simulink model "StewartPlatform"  (R2020a)
settings: Solver=VariableStepAuto  StartTime=0.1  StopTime=35  FixedStep=0.01  MaxStep=0.01  RelTol=1e-3  EnableMultiTasking=on
values from neighbouring files (symbols this model uses):
  Arm_Wrap = 0.75    [ParamLibrary.sldd]
  BaseArm_Wrap = 0.6    [ParamLibrary.sldd]
undefined symbols (not defined in the file or in its folder): X, Y, Z
libraries: sm_lib x122, nesl_utility x32
(part 5 of 5)

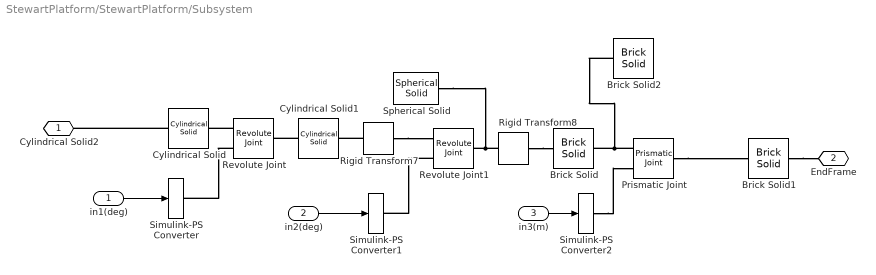
== system StewartPlatform/StewartPlatform/Subsystem ==
  in1(deg) : Inport
  in2(deg) : Inport  Port=2
  in3(m) : Inport  Port=3
  Brick Solid : sm_lib/Body Elements/Brick Solid  GraphicAmbientColor=[0.15 0.15 0.15 1.0]  BasedOnType=Density  BrickDimensions=[0.1 0.05 0.5]  BrickDimensionUnits=m  CenterOfMass=[0 0 0]  CenterOfMassUnits=m  GraphicDiffuseColor=[0.5 0.5 0.5]  Density=1000  DensityUnits=kg/m^3  DoExposeReferenceFrame=off  GraphicEmissiveColor=[0.0 0.0 0.0 1.0]  ExportEntireGeometry=off  SerializedFrames=<Frames><Frame><Id>Frame1</Id><Value><Name>F1</Name><Origin><Source>GeometricFeature</Source><FeatureName>-z surface</FeatureName></Origin><PrimaryAxis><DefinedDirection>+Z</DefinedDirection><Source>ReferenceFrame</Source><SourceDirection>+Z</SourceDirection><FeatureName></FeatureName></PrimaryAxis><SecondaryAxis><DefinedDirection>+X</DefinedDirection><Source>ReferenceFrame</Source><SourceDirection>+X</SourceDirection><FeatureName></FeatureName></SecondaryAxis></Value></Frame><Frame><Id>Frame2</Id><Value><Name>F2</Name><Origin><Source>GeometricFeature</Source><FeatureName>+z surface</FeatureName></Origin><PrimaryAxis><DefinedDirection>+Z</DefinedDirection><Source>ReferenceFrame</Source><SourceDirection>+Z</SourceDirection><FeatureName></FeatureName></PrimaryAxis><SecondaryAxis><DefinedDirection>+X</DefinedDirection><Source>ReferenceFrame</Source><SourceDirection>+X</SourceDirection><FeatureName></FeatureName></SecondaryAxis></Value></Frame></Frames>  MarkerShape=Sphere  MarkerSize=10  GraphicType=FromGeometry  InertiaType=CalculateFromGeometry  Mass=1  MassUnits=kg  MomentsOfInertia=[1 1 1]  MomentsOfInertiaUnits=kg*m^2  GraphicOpacity=1.0  ProductsOfInertia=[0 0 0]  ProductsOfInertiaUnits=kg*m^2  GraphicShininess=75  GraphicSpecularColor=[0.5 0.5 0.5 1.0]  GraphicVisPropType=SimpleVisualProperties
  Brick Solid1 : sm_lib/Body Elements/Brick Solid  GraphicAmbientColor=[0.15 0.15 0.15 1.0]  BasedOnType=Density  BrickDimensions=[0.075 0.02 1]  BrickDimensionUnits=m  CenterOfMass=[0 0 0]  CenterOfMassUnits=m  GraphicDiffuseColor=[0.5 0.5 0.5]  Density=1000  DensityUnits=kg/m^3  DoExposeReferenceFrame=off  GraphicEmissiveColor=[0.0 0.0 0.0 1.0]  ExportEntireGeometry=off  SerializedFrames=<Frames><Frame><Id>Frame1</Id><Value><Name>F1</Name><Origin><Source>GeometricFeature</Source><FeatureName>-z surface</FeatureName></Origin><PrimaryAxis><DefinedDirection>+Z</DefinedDirection><Source>ReferenceFrame</Source><SourceDirection>+Z</SourceDirection><FeatureName></FeatureName></PrimaryAxis><SecondaryAxis><DefinedDirection>+X</DefinedDirection><Source>ReferenceFrame</Source><SourceDirection>+X</SourceDirection><FeatureName></FeatureName></SecondaryAxis></Value></Frame><Frame><Id>Frame2</Id><Value><Name>F2</Name><Origin><Source>GeometricFeature</Source><FeatureName>+z surface</FeatureName></Origin><PrimaryAxis><DefinedDirection>+Z</DefinedDirection><Source>ReferenceFrame</Source><SourceDirection>+Z</SourceDirection><FeatureName></FeatureName></PrimaryAxis><SecondaryAxis><DefinedDirection>+X</DefinedDirection><Source>ReferenceFrame</Source><SourceDirection>+X</SourceDirection><FeatureName></FeatureName></SecondaryAxis></Value></Frame></Frames>  MarkerShape=Sphere  MarkerSize=10  GraphicType=FromGeometry  InertiaType=CalculateFromGeometry  Mass=1  MassUnits=kg  MomentsOfInertia=[1 1 1]  MomentsOfInertiaUnits=kg*m^2  GraphicOpacity=1.0  ProductsOfInertia=[0 0 0]  ProductsOfInertiaUnits=kg*m^2  GraphicShininess=75  GraphicSpecularColor=[0.5 0.5 0.5 1.0]  GraphicVisPropType=SimpleVisualProperties
  Brick Solid2 : sm_lib/Body Elements/Brick Solid  GraphicAmbientColor=[0.15 0.15 0.15 1.0]  BasedOnType=Density  BrickDimensions=[0.1 0.05 1.5]  BrickDimensionUnits=m  CenterOfMass=[0 0 0]  CenterOfMassUnits=m  GraphicDiffuseColor=[0.5 0.5 0.5]  Density=1000  DensityUnits=kg/m^3  DoExposeReferenceFrame=off  GraphicEmissiveColor=[0.0 0.0 0.0 1.0]  ExportEntireGeometry=off  SerializedFrames=<Frames><Frame><Id>Frame1</Id><Value><Name>F1</Name><Origin><Source>GeometricFeature</Source><FeatureName>-z surface</FeatureName></Origin><PrimaryAxis><DefinedDirection>+Z</DefinedDirection><Source>ReferenceFrame</Source><SourceDirection>+Z</SourceDirection><FeatureName></FeatureName></PrimaryAxis><SecondaryAxis><DefinedDirection>+X</DefinedDirection><Source>ReferenceFrame</Source><SourceDirection>+X</SourceDirection><FeatureName></FeatureName></SecondaryAxis></Value></Frame></Frames>  MarkerShape=Sphere  MarkerSize=10  GraphicType=FromGeometry  InertiaType=CalculateFromGeometry  Mass=1  MassUnits=kg  MomentsOfInertia=[1 1 1]  MomentsOfInertiaUnits=kg*m^2  GraphicOpacity=1.0  ProductsOfInertia=[0 0 0]  ProductsOfInertiaUnits=kg*m^2  GraphicShininess=75  GraphicSpecularColor=[0.5 0.5 0.5 1.0]  GraphicVisPropType=SimpleVisualProperties
  Cylindrical Solid : sm_lib/Body Elements/Cylindrical Solid  GraphicAmbientColor=[0.15 0.15 0.15 1.0]  BasedOnType=Density  CenterOfMass=[0 0 0]  CenterOfMassUnits=m  GraphicDiffuseColor=[0.5 0.5 0.5]  CylinderLength=0.2  CylinderLengthUnits=m  CylinderRadius=0.3  CylinderRadiusUnits=m  Density=1000  DensityUnits=kg/m^3  DoExposeReferenceFrame=off  GraphicEmissiveColor=[0.0 0.0 0.0 1.0]  ExportEntireGeometry=off  SerializedFrames=<Frames><Frame><Id>Frame1</Id><Value><Name>F1</Name><Origin><Source>GeometricFeature</Source><FeatureName>bottom surface</FeatureName></Origin><PrimaryAxis><DefinedDirection>+Z</DefinedDirection><Source>ReferenceFrame</Source><SourceDirection>+Z</SourceDirection><FeatureName></FeatureName></PrimaryAxis><SecondaryAxis><DefinedDirection>+X</DefinedDirection><Source>ReferenceFrame</Source><SourceDirection>+X</SourceDirection><FeatureName></FeatureName></SecondaryAxis></Value></Frame><Frame><Id>Frame2</Id><Value><Name>F2</Name><Origin><Source>GeometricFeature</Source><FeatureName>top surface</FeatureName></Origin><PrimaryAxis><DefinedDirection>+Z</DefinedDirection><Source>ReferenceFrame</Source><SourceDirection>+Z</SourceDirection><FeatureName></FeatureName></PrimaryAxis><SecondaryAxis><DefinedDirection>+X</DefinedDirection><Source>ReferenceFrame</Source><SourceDirection>+X</SourceDirection><FeatureName></FeatureName></SecondaryAxis></Value></Frame></Frames>  MarkerShape=Sphere  MarkerSize=10  GraphicType=FromGeometry  InertiaType=CalculateFromGeometry  Mass=1  MassUnits=kg  MomentsOfInertia=[1 1 1]  MomentsOfInertiaUnits=kg*m^2  GraphicOpacity=1.0  ProductsOfInertia=[0 0 0]  ProductsOfInertiaUnits=kg*m^2  GraphicShininess=75  GraphicSpecularColor=[0.5 0.5 0.5 1.0]  GraphicVisPropType=SimpleVisualProperties
  Cylindrical Solid1 : sm_lib/Body Elements/Cylindrical Solid  GraphicAmbientColor=[0.15 0.15 0.15 1.0]  BasedOnType=Density  CenterOfMass=[0 0 0]  CenterOfMassUnits=m  GraphicDiffuseColor=[0.5 0.5 0.5]  CylinderLength=0.4  CylinderLengthUnits=m  CylinderRadius=0.1  CylinderRadiusUnits=m  Density=1000  DensityUnits=kg/m^3  DoExposeReferenceFrame=off  GraphicEmissiveColor=[0.0 0.0 0.0 1.0]  ExportEntireGeometry=off  SerializedFrames=<Frames><Frame><Id>Frame1</Id><Value><Name>F1</Name><Origin><Source>GeometricFeature</Source><FeatureName>bottom surface</FeatureName></Origin><PrimaryAxis><DefinedDirection>+Z</DefinedDirection><Source>ReferenceFrame</Source><SourceDirection>+Z</SourceDirection><FeatureName></FeatureName></PrimaryAxis><SecondaryAxis><DefinedDirection>+X</DefinedDirection><Source>ReferenceFrame</Source><SourceDirection>+X</SourceDirection><FeatureName></FeatureName></SecondaryAxis></Value></Frame><Frame><Id>Frame2</Id><Value><Name>F2</Name><Origin><Source>GeometricFeature</Source><FeatureName>top surface</FeatureName></Origin><PrimaryAxis><DefinedDirection>+Z</DefinedDirection><Source>ReferenceFrame</Source><SourceDirection>+Z</SourceDirection><FeatureName></FeatureName></PrimaryAxis><SecondaryAxis><DefinedDirection>+X</DefinedDirection><Source>ReferenceFrame</Source><SourceDirection>+X</SourceDirection><FeatureName></FeatureName></SecondaryAxis></Value></Frame></Frames>  MarkerShape=Sphere  MarkerSize=10  GraphicType=FromGeometry  InertiaType=CalculateFromGeometry  Mass=1  MassUnits=kg  MomentsOfInertia=[1 1 1]  MomentsOfInertiaUnits=kg*m^2  GraphicOpacity=1.0  ProductsOfInertia=[0 0 0]  ProductsOfInertiaUnits=kg*m^2  GraphicShininess=75  GraphicSpecularColor=[0.5 0.5 0.5 1.0]  GraphicVisPropType=SimpleVisualProperties
  Prismatic Joint : sm_lib/Joints/Prismatic Joint  JointMode=Normal  SenseConstraintForce=off  SenseConstraintForceX=off  SenseConstraintForceY=off  SenseConstraintForceZ=off  SenseConstraintTorque=off  SenseConstraintTorqueX=off  SenseConstraintTorqueY=off  SenseConstraintTorqueZ=off  SenseTotalForce=off  SenseTotalForceX=off  SenseTotalForceY=off  SenseTotalForceZ=off  SenseTotalTorque=off  SenseTotalTorqueX=off  SenseTotalTorqueY=off  SenseTotalTorqueZ=off  CompositeWrenchDir=FollowerOnBase  CompositeWrenchFrame=BaseFrame  EquilibriumPosition=0  EquilibriumPositionUnits=m  SpringStiffness=0  SpringStiffnessUnits=N/m  DampingCoefficient=0  DampingCoefficientUnits=N/(m/s)  TorqueActuationMode=ComputedTorque  MotionActuationMode=InputMotion  SensePosition=off  SenseVelocity=off  SenseAcceleration=off  SenseTorqueForce=off  SenseLowerLimitTorqueForce=off  SenseUpperLimitTorqueForce=off  LowerLimitSpecify=on  LowerLimitBound=Arm_LowLimit  LowerLimitBoundUnits=m  LowerLimitStiffness=1e6  LowerLimitStiffnessUnits=N/m  LowerLimitDamping=1e3  LowerLimitDampingUnits=N/(m/s)  LowerLimitTransitionRegionWidth=1e-4  LowerLimitTransitionRegionWidthUnits=m  UpperLimitSpecify=on  UpperLimitBound=Arm_HighLimit  UpperLimitBoundUnits=m  UpperLimitStiffness=1e6  UpperLimitStiffnessUnits=N/m  UpperLimitDamping=1e3  UpperLimitDampingUnits=N/(m/s)  UpperLimitTransitionRegionWidth=1e-4  UpperLimitTransitionRegionWidthUnits=m  PositionTargetSpecify=off  PositionTargetPriority=Low  PositionTargetValue=0.8  PositionTargetValueUnits=m  VelocityTargetSpecify=off  VelocityTargetPriority=High  VelocityTargetValue=0  VelocityTargetValueUnits=m/s
  Revolute Joint : sm_lib/Joints/Revolute Joint  JointMode=Normal  SenseConstraintForce=off  SenseConstraintForceX=off  SenseConstraintForceY=off  SenseConstraintForceZ=off  SenseConstraintTorque=off  SenseConstraintTorqueX=off  SenseConstraintTorqueY=off  SenseConstraintTorqueZ=off  SenseTotalForce=off  SenseTotalForceX=off  SenseTotalForceY=off  SenseTotalForceZ=off  SenseTotalTorque=off  SenseTotalTorqueX=off  SenseTotalTorqueY=off  SenseTotalTorqueZ=off  CompositeWrenchDir=FollowerOnBase  CompositeWrenchFrame=BaseFrame  EquilibriumPosition=0  EquilibriumPositionUnits=deg  SpringStiffness=0  SpringStiffnessUnits=N*m/deg  DampingCoefficient=0  DampingCoefficientUnits=N*m/(deg/s)  TorqueActuationMode=ComputedTorque  MotionActuationMode=InputMotion  SensePosition=off  SenseVelocity=off  SenseAcceleration=off  SenseTorqueForce=off  SenseLowerLimitTorqueForce=off  SenseUpperLimitTorqueForce=off  LowerLimitSpecify=off  LowerLimitBound=-90  LowerLimitBoundUnits=deg  LowerLimitStiffness=1e4  LowerLimitStiffnessUnits=N*m/deg  LowerLimitDamping=10  LowerLimitDampingUnits=N*m/(deg/s)  LowerLimitTransitionRegionWidth=0.1  LowerLimitTransitionRegionWidthUnits=deg  UpperLimitSpecify=off  UpperLimitBound=90  UpperLimitBoundUnits=deg  UpperLimitStiffness=1e4  UpperLimitStiffnessUnits=N*m/deg  UpperLimitDamping=10  UpperLimitDampingUnits=N*m/(deg/s)  UpperLimitTransitionRegionWidth=0.1  UpperLimitTransitionRegionWidthUnits=deg  PositionTargetSpecify=off  PositionTargetPriority=High  PositionTargetValue=0  PositionTargetValueUnits=deg  VelocityTargetSpecify=off  VelocityTargetPriority=High  VelocityTargetValue=0  VelocityTargetValueUnits=deg/s
  Revolute Joint1 : sm_lib/Joints/Revolute Joint  JointMode=Normal  SenseConstraintForce=off  SenseConstraintForceX=off  SenseConstraintForceY=off  SenseConstraintForceZ=off  SenseConstraintTorque=off  SenseConstraintTorqueX=off  SenseConstraintTorqueY=off  SenseConstraintTorqueZ=off  SenseTotalForce=off  SenseTotalForceX=off  SenseTotalForceY=off  SenseTotalForceZ=off  SenseTotalTorque=off  SenseTotalTorqueX=off  SenseTotalTorqueY=off  SenseTotalTorqueZ=off  CompositeWrenchDir=FollowerOnBase  CompositeWrenchFrame=BaseFrame  EquilibriumPosition=0  EquilibriumPositionUnits=deg  SpringStiffness=0  SpringStiffnessUnits=N*m/deg  DampingCoefficient=0  DampingCoefficientUnits=N*m/(deg/s)  TorqueActuationMode=ComputedTorque  MotionActuationMode=InputMotion  SensePosition=off  SenseVelocity=off  SenseAcceleration=off  SenseTorqueForce=off  SenseLowerLimitTorqueForce=off  SenseUpperLimitTorqueForce=off  LowerLimitSpecify=off  LowerLimitBound=-90  LowerLimitBoundUnits=deg  LowerLimitStiffness=1e4  LowerLimitStiffnessUnits=N*m/deg  LowerLimitDamping=10  LowerLimitDampingUnits=N*m/(deg/s)  LowerLimitTransitionRegionWidth=0.1  LowerLimitTransitionRegionWidthUnits=deg  UpperLimitSpecify=off  UpperLimitBound=90  UpperLimitBoundUnits=deg  UpperLimitStiffness=1e4  UpperLimitStiffnessUnits=N*m/deg  UpperLimitDamping=10  UpperLimitDampingUnits=N*m/(deg/s)  UpperLimitTransitionRegionWidth=0.1  UpperLimitTransitionRegionWidthUnits=deg  PositionTargetSpecify=off  PositionTargetPriority=High  PositionTargetValue=0  PositionTargetValueUnits=deg  VelocityTargetSpecify=off  VelocityTargetPriority=High  VelocityTargetValue=0  VelocityTargetValueUnits=deg/s
  Rigid Transform7 : sm_lib/Frames and Transforms/Rigid Transform  TranslationMethod=None  TranslationStandardOffset=0  TranslationLengthUnit=m  TranslationStandardAxis=+Z  TranslationCartesianOffset=[0 0 0]  TranslationROffset=1  TranslationROffsetUnits=m  TranslationZOffset=0  TranslationZOffsetUnits=m  TranslationThetaOffset=0  TranslationThetaOffsetUnits=deg  RotationMethod=StandardAxis  RotationAngleUnits=deg  RotationStandardAxis=+Y  RotationAngle=90.0  RotationArbitraryAxis=[0 0 1]  FollAlignAxisA=+X  BaseAlignAxisA=+Y  FollAlignAxisB=+Y  BaseAlignAxisB=+Z  RotationSequenceAxes=FollowerAxes  RotationSequence=XYX  RotationSequenceAngles=[0 0 0]  RotationSequenceAnglesUnits=deg  RotationMatrix=[1 0 0; 0 1 0; 0 0 1]
  Rigid Transform8 : sm_lib/Frames and Transforms/Rigid Transform  TranslationMethod=None  TranslationStandardOffset=0  TranslationLengthUnit=m  TranslationStandardAxis=+Z  TranslationCartesianOffset=[0 0 0]  TranslationROffset=1  TranslationROffsetUnits=m  TranslationZOffset=0  TranslationZOffsetUnits=m  TranslationThetaOffset=0  TranslationThetaOffsetUnits=deg  RotationMethod=StandardAxis  RotationAngleUnits=deg  RotationStandardAxis=+Y  RotationAngle=90.0  RotationArbitraryAxis=[0 0 1]  FollAlignAxisA=+X  BaseAlignAxisA=+Y  FollAlignAxisB=+Y  BaseAlignAxisB=+Z  RotationSequenceAxes=FollowerAxes  RotationSequence=XYX  RotationSequenceAngles=[0 0 0]  RotationSequenceAnglesUnits=deg  RotationMatrix=[1 0 0; 0 1 0; 0 0 1]
  Simulink-PS Converter : nesl_utility/Simulink-PS Converter  PhysicalDomain=network_engine_domain  SubClassName=ps_input  LeftPortType=input  RightPortType=output  PseudoPeriodic=off  Frequencies=[]  NoiseDistribution=none  NoiseParameters=[]  Unit=1  AffineConversion=off  FilteringAndDerivatives=filter  SimscapeFilterOrder=2  InputFilterTimeConstant=0.001  UdotUserProvided=0
  Simulink-PS Converter1 : nesl_utility/Simulink-PS Converter  PhysicalDomain=network_engine_domain  SubClassName=ps_input  LeftPortType=input  RightPortType=output  PseudoPeriodic=off  Frequencies=[]  NoiseDistribution=none  NoiseParameters=[]  Unit=1  AffineConversion=off  FilteringAndDerivatives=filter  SimscapeFilterOrder=2  InputFilterTimeConstant=0.001  UdotUserProvided=0
  Simulink-PS Converter2 : nesl_utility/Simulink-PS Converter  PhysicalDomain=network_engine_domain  SubClassName=ps_input  LeftPortType=input  RightPortType=output  PseudoPeriodic=off  Frequencies=[]  NoiseDistribution=none  NoiseParameters=[]  Unit=1  AffineConversion=off  FilteringAndDerivatives=filter  SimscapeFilterOrder=2  InputFilterTimeConstant=0.001  UdotUserProvided=0
  Spherical Solid : sm_lib/Body Elements/Spherical Solid  GraphicAmbientColor=[0.15 0.15 0.15 1.0]  BasedOnType=Density  CenterOfMass=[0 0 0]  CenterOfMassUnits=m  GraphicDiffuseColor=[0.5 0.5 0.5]  Density=1000  DensityUnits=kg/m^3  DoExposeReferenceFrame=on  GraphicEmissiveColor=[0.0 0.0 0.0 1.0]  ExportEntireGeometry=off  SerializedExposedGeometries=<ExposedGeometries/>  SerializedFrames=<Frames/>  MarkerShape=Sphere  MarkerSize=10  GraphicType=FromGeometry  InertiaType=CalculateFromGeometry  Mass=1  MassUnits=kg  MomentsOfInertia=[1 1 1]  MomentsOfInertiaUnits=kg*m^2  GraphicOpacity=1.0  ProductsOfInertia=[0 0 0]  ProductsOfInertiaUnits=kg*m^2  GraphicShininess=75  GraphicSpecularColor=[0.5 0.5 0.5 1.0]  SphereRadius=0.1  SphereRadiusUnits=m  GraphicVisPropType=SimpleVisualProperties
  Cylindrical Solid2 : PMIOPort  Side=Left
  EndFrame : PMIOPort  Port=2  Side=Right
  wires:
  in1(deg)/1 -> Simulink-PS Converter/1
  in2(deg)/1 -> Simulink-PS Converter1/1
  in3(m)/1 -> Simulink-PS Converter2/1
  connections:
  Prismatic Joint/LConn1 -- Brick Solid2/LConn1 -- Brick Solid/RConn1
  Rigid Transform7/RConn1 -- Revolute Joint1/LConn1
  Rigid Transform7/LConn1 -- Cylindrical Solid1/RConn1
  Rigid Transform8/LConn1 -- Spherical Solid/RConn1 -- Revolute Joint1/RConn1
  Cylindrical Solid1/LConn1 -- Revolute Joint/RConn1
  Revolute Joint/LConn1 -- Cylindrical Solid/RConn1
  Rigid Transform8/RConn1 -- Brick Solid/LConn1
  Revolute Joint/LConn2 -- Simulink-PS Converter/RConn1
  Revolute Joint1/LConn2 -- Simulink-PS Converter1/RConn1
  Prismatic Joint/RConn1 -- Brick Solid1/LConn1
  Cylindrical Solid/LConn1 -- Cylindrical Solid2/RConn1
  Simulink-PS Converter2/RConn1 -- Prismatic Joint/LConn2
  Brick Solid1/RConn1 -- EndFrame/RConn1

== matlab function StewartPlatform/MATLAB Function1 ==
  data: TF_CA input; alpha output; beita output; dL output
function [alpha,beita,dL] = fcn(TF_CA)
% 原有计算逻辑
TF_CEnd_Static = [1,0.004,0.1,0.17;
                  0.1,-0.07,-1,-1.77;
                  0.0026,1,-0.07,4;
                  0,0,0,1];
L = 0.6;
L1 = 0.5;
L2 = 1;
TF_AEnd = pinv(TF_CA) * TF_CEnd_Static;
x = TF_AEnd(1,4);
y = TF_AEnd(2,4);
z = TF_AEnd(3,4);

dL = sqrt((z-L)^2 + x^2 + y^2) - (L1 + L2); % 更安全的sqrt写法
beita = asin((z-L)/(L1+L2+dL));
alpha = asin(y/( (L1+L2+dL)*cos(beita) )); % 修正分母的括号
end

== matlab function StewartPlatform/TF_Coder ==
  data: RotationMatrix input; X input; TF_Matrix output; Y input; Z input
function TF_Matrix = fcn(RotationMatrix,X, Y, Z)
 T = [
        RotationMatrix(1,1), RotationMatrix(1,2), RotationMatrix(1,3), X;
        RotationMatrix(2,1), RotationMatrix(2,2), RotationMatrix(2,3), Y;
        RotationMatrix(3,1), RotationMatrix(3,2), RotationMatrix(3,3), Z;
        0, 0, 0, 1;
    ];

TF_Matrix = T;

== matlab function StewartPlatform/TF_Coder1 ==
  data: RotationMatrix input; X input; TF_Matrix output; Y input; Z input
function TF_Matrix = fcn(RotationMatrix,X, Y, Z)
 T = [
        RotationMatrix(1,1), RotationMatrix(1,2), RotationMatrix(1,3), X;
        RotationMatrix(2,1), RotationMatrix(2,2), RotationMatrix(2,3), Y;
        RotationMatrix(3,1), RotationMatrix(3,2), RotationMatrix(3,3), Z;
        0, 0, 0, 1;
    ];

TF_Matrix = T;

== matlab function StewartPlatform/TF_Coder ==
  data: RotationMatrix input; X input; TF_Matrix output; Y input; Z input
function TF_Matrix = fcn(RotationMatrix,X, Y, Z)
 T = [
        RotationMatrix(1,1), RotationMatrix(1,2), RotationMatrix(1,3), X;
        RotationMatrix(2,1), RotationMatrix(2,2), RotationMatrix(2,3), Y;
        RotationMatrix(3,1), RotationMatrix(3,2), RotationMatrix(3,3), Z;
        0, 0, 0, 1;
    ];

TF_Matrix = T;

== matlab function StewartPlatform/Controller_SelfFit ==
  data: TF_CB input; TF_BA input; Arm1 output; Arm2 output; Arm3 output; Arm4 output; Arm5 output; Arm6 output; Mode input; Robustness input
function [Arm1, Arm2, Arm3, Arm4, Arm5, Arm6] = fcn(TF_CB,TF_BA,Mode,Robustness)
%Frame_A相对Frame_B初始位姿
TF_BA_Static = [
-0.866  ,-0.5    ,0     ,0 ;    
 0.5    ,-0.866  ,0     ,0 ;
 0      ,0       ,1     ,1.518;
 0      ,0       ,0     ,1    
];
%Frame_B相对Frame_C初始位姿
TF_CB_Static = [
0.866  ,-0.5    ,0     ,0 ;    
 0.5    ,0.866  ,0     ,0 ;
 0      ,0       ,1     ,(1.305+0.6);
 0      ,0       ,0     ,1    
];
TF_CA_Static = TF_CB_Static * TF_BA_Static ;
%A面和B面点坐标
Ra = 0.8;
a1 = [-Ra/2 ; -(3)^(0.5)*Ra/2 ; 0];
a2 = [Ra ; 0 ; 0];
a3 = [-Ra/2 ; (3)^(0.5)*Ra/2 ; 0 ];
Rb = 1;
b1 = [Rb;0;0];
b2 = [Rb/2;(3)^(0.5)*Rb/2;0];
b3 = [-Rb/2;(3)^(0.5)*Rb/2;0];
b4 = [-Rb;0;0];
b5 = [-Rb/2;-(3)^(0.5)*Rb/2;0];
b6 = [Rb/2;-(3)^(0.5)*Rb/2;0];
if Mode == 0
%%上平台完全静止
%求解最上层平台Frame_A相对Frame_B的目标位姿
    TF_BA_Target = pinv(TF_CB) * TF_CA_Static ;
    Arm1 = norm( TF_BA_Target*[a1;1] - [b1;1]  ) - 1.6;
    Arm2 = norm( TF_BA_Target*[a1;1] - [b2;1]  ) - 1.6;
    Arm3 = norm( TF_BA_Target*[a2;1] - [b3;1]  ) - 1.6;
    Arm4 = norm( TF_BA_Target*[a2;1] - [b4;1]  ) - 1.6;
    Arm5 = norm( TF_BA_Target*[a3;1] - [b5;1]  ) - 1.6;
    Arm6 = norm( TF_BA_Target*[a3;1] - [b6;1]  ) - 1.6;
%%上平台自由平滑跟随
elseif Mode == 1
    TF_CA_NOW = TF_CB * TF_BA;
    TF_CA_Target = [
        TF_CA_Static(1,1) , TF_CA_Static(1,2) , TF_CA_Static(1,3) , (TF_CA_Static(1,4)*Robustness + TF_CA_NOW(1,4))/(Robustness+1);
        TF_CA_Static(2,1) , TF_CA_Static(2,2) , TF_CA_Static(2,3) , (TF_CA_Static(2,4)*Robustness + TF_CA_NOW(2,4))/(Robustness+1) ;
        TF_CA_Static(3,1) , TF_CA_Static(3,2) , TF_CA_Static(3,3) , (TF_CA_Static(3,4)*Robustness + TF_CA_NOW(3,4))/(Robustness+1);
        0 ,0 ,0 ,1
    ];
    TF_BA_Target = pinv(TF_CB) * TF_CA_Target;
    Arm1 = norm( TF_BA_Target*[a1;1] - [b1;1]  ) - 1.6;
    Arm2 = norm( TF_BA_Target*[a1;1] - [b2;1]  ) - 1.6;
    Arm3 = norm( TF_BA_Target*[a2;1] - [b3;1]  ) - 1.6;
    Arm4 = norm( TF_BA_Target*[a2;1] - [b4;1]  ) - 1.6;
    Arm5 = norm( TF_BA_Target*[a3;1] - [b5;1]  ) - 1.6;
    Arm6 = norm( TF_BA_Target*[a3;1] - [b6;1]  ) - 1.6;
    
else
Arm1 = 0;
Arm2 = 0;
Arm3 = 0;
Arm4 = 0;
Arm5 = 0;
Arm6 = 0;
end

end

== matlab function StewartPlatform/TF_Coder1 ==
  data: RotationMatrix input; X input; TF_Matrix output; Y input; Z input
function TF_Matrix = fcn(RotationMatrix,X, Y, Z)
 T = [
        RotationMatrix(1,1), RotationMatrix(1,2), RotationMatrix(1,3), X;
        RotationMatrix(2,1), RotationMatrix(2,2), RotationMatrix(2,3), Y;
        RotationMatrix(3,1), RotationMatrix(3,2), RotationMatrix(3,3), Z;
        0, 0, 0, 1;
    ];

TF_Matrix = T;

== matlab function StewartPlatform/Controller_outctrl ==
  data: TF_CB input; Arm1 output; TF_BA input; TF_CA_Static_last input; clock input; Mode input; Arm2 output; Arm3 output; Arm4 output; Arm5 output; Arm6 output; Robustness input; M11 output; M12 output; M13 output; M14 output; M21 output; M22 output; M23 output; M24 output; M31 output; M32 output; M33 output; M34 output
function [Arm1, Arm2, Arm3, Arm4, Arm5, Arm6, M11, M12, M13, M14, M21, M22, M23, M24, M31, M32, M33, M34]  = fcn(TF_CB,TF_BA,TF_CA_Static_last,clock,Mode,Robustness)
%Frame_A相对Frame_B初始位姿
TF_BA_Static = [
-0.866  ,-0.5    ,0     ,0 ;    
 0.5    ,-0.866  ,0     ,0 ;
 0      ,0       ,1     ,1.518;
 0      ,0       ,0     ,1    
];
%Frame_B相对Frame_C初始位姿
TF_CB_Static = [
0.866  ,-0.5    ,0     ,0 ;    
 0.5    ,0.866  ,0     ,0 ;
 0      ,0       ,1     ,(1.305+0.6);
 0      ,0       ,0     ,1    
];
TF_CA_Static = TF_CB_Static * TF_BA_Static ;
%继承上一周期的TF_CA_Static
start_time = 1;
phase = 2;
if clock > start_time
    TF_CA_Static = TF_CA_Static_last;
end

seta = 0.002;
TF_ROT_X = [1,0,0,0;
            0,cos(seta),-sin(seta),0;
            0,sin(seta),cos(seta),0;
            0,0,0,1];
TF_ROT_X_n = [1,0,0,0;
            0,cos(-seta),-sin(-seta),0;
            0,sin(-seta),cos(-seta),0;
            0,0,0,1];
TF_ROT_Y = [cos(seta), 0, sin(seta), 0;
            0, 1, 0, 0;
            -sin(seta), 0, cos(seta), 0;
            0, 0, 0, 1];
TF_ROT_Y_n = [cos(-seta),0,sin(-seta),0;
            0,1,0,0;
            -sin(-seta),0,cos(-seta),0;
            0,0,0,1];
TF_ROT_Z = [cos(seta),-sin(seta),0,0;
            sin(seta),cos(seta),0,0;
            0,0,1,0;
            0,0,0,1;
];
TF_ROT_Z_n = [cos(-seta),-sin(-seta),0,0;
            sin(-seta),cos(-seta),0,0;
            0,0,1,0;
            0,0,0,1;
];
%x轴倾斜
if (start_time<clock)&&(clock<start_time+phase)
    TF_CA_Static = TF_CA_Static * TF_ROT_X_n;   
end
if (start_time+phase<clock)&&(clock<start_time+2*phase)
    TF_CA_Static =  TF_CA_Static * TF_ROT_X;   
end
if (start_time+2*phase<clock)&&(clock<start_time+3*phase)
    TF_CA_Static = TF_CA_Static * TF_ROT_X;   
end
if (start_time+3*phase<clock)&&(clock<start_time+4*phase)
    TF_CA_Static = TF_CA_Static * TF_ROT_X_n;   
end
%y轴倾斜
if (start_time+4*phase<clock)&&(clock<start_time+5*phase)
    TF_CA_Static = TF_CA_Static * TF_ROT_Y_n;   
end
if (start_time+5*phase<clock)&&(clock<start_time+6*phase)
    TF_CA_Static = TF_CA_Static * TF_ROT_Y;   
end
if (start_time+6*phase<clock)&&(clock<start_time+7*phase)
    TF_CA_Static = TF_CA_Static * TF_ROT_Y;   
end
if (start_time+7*phase<clock)&&(clock<start_time+8*phase)
    TF_CA_Static = TF_CA_Static * TF_ROT_Y_n;   
end
%z轴倾斜
if (start_time+8*phase<clock)&&(clock<start_time+9*phase)
    TF_CA_Static = TF_CA_Static * TF_ROT_Z_n;   
end
if (start_time+9*phase<clock)&&(clock<start_time+10*phase)
    TF_CA_Static = TF_CA_Static * TF_ROT_Z;   
end
if (start_time+10*phase<clock)&&(clock<start_time+11*phase)
    TF_CA_Static = TF_CA_Static * TF_ROT_Z;   
end
if (start_time+11*phase<clock)&&(clock<start_time+12*phase)
    TF_CA_Static = TF_CA_Static * TF_ROT_Z_n;   
end


%A面和B面点坐标
Ra = 0.8;
a1 = [-Ra/2 ; -(3)^(0.5)*Ra/2 ; 0];
a2 = [Ra ; 0 ; 0];
a3 = [-Ra/2 ; (3)^(0.5)*Ra/2 ; 0 ];
Rb = 1;
b1 = [Rb;0;0];
b2 = [Rb/2;(3)^(0.5)*Rb/2;0];
b3 = [-Rb/2;(3)^(0.5)*Rb/2;0];
b4 = [-Rb;0;0];
b5 = [-Rb/2;-(3)^(0.5)*Rb/2;0];
b6 = [Rb/2;-(3)^(0.5)*Rb/2;0];
if Mode == 1
    TF_CA_NOW = TF_CB * TF_BA;
    TF_CA_Target = [
        TF_CA_Static(1,1) , TF_CA_Static(1,2) , TF_CA_Static(1,3) , (TF_CA_Static(1,4)*Robustness + TF_CA_NOW(1,4))/(Robustness+1);
        TF_CA_Static(2,1) , TF_CA_Static(2,2) , TF_CA_Static(2,3) , (TF_CA_Static(2,4)*Robustness + TF_CA_NOW(2,4))/(Robustness+1) ;
        TF_CA_Static(3,1) , TF_CA_Static(3,2) , TF_CA_Static(3,3) , (TF_CA_Static(3,4)*Robustness + TF_CA_NOW(3,4))/(Robustness+1);
        0 ,0 ,0 ,1
    ];
    TF_BA_Target = pinv(TF_CB) * TF_CA_Target;
    Arm1 = norm( TF_BA_Target*[a1;1] - [b1;1]  ) - 1.6;
    Arm2 = norm( TF_BA_Target*[a1;1] - [b2;1]  ) - 1.6;
    Arm3 = norm( TF_BA_Target*[a2;1] - [b3;1]  ) - 1.6;
    Arm4 = norm( TF_BA_Target*[a2;1] - [b4;1]  ) - 1.6;
    Arm5 = norm( TF_BA_Target*[a3;1] - [b5;1]  ) - 1.6;
    Arm6 = norm( TF_BA_Target*[a3;1] - [b6;1]  ) - 1.6; 

else
Arm1 = 0;
Arm2 = 0;
Arm3 = 0;
Arm4 = 0;
Arm5 = 0;
Arm6 = 0;

end
TF_CA_Static_latest = TF_CA_Static;
M11 = TF_CA_Static_latest(1,1);
M12 = TF_CA_Static_latest(1,2);
M13 = TF_CA_Static_latest(1,3);
M14 = TF_CA_Static_latest(1,4);
M21 = TF_CA_Static_latest(2,1);
M22 = TF_CA_Static_latest(2,2);
M23 = TF_CA_Static_latest(2,3);
M24 = TF_CA_Static_latest(2,4);
M31 = TF_CA_Static_latest(3,1);
M32 = TF_CA_Static_latest(3,2);
M33 = TF_CA_Static_latest(3,3);
M34 = TF_CA_Static_latest(3,4);


end

== matlab function StewartPlatform/MATLAB Function ==
  data: M11 input; TF_Matrix output; M12 input; M13 input; M14 input; M21 input; M22 input; M23 input; M24 input; M31 input; M32 input; M33 input; M34 input
function TF_Matrix = fcn(M11, M12, M13, M14, M21, M22, M23, M24, M31, M32, M33, M34)
TF_Matrix = [
M11, M12, M13, M14;
M21, M22, M23, M24;
M31, M32, M33, M34;
0, 0, 0, 1
];
